simulink model "core_attitude"  (R2022b)
settings: Solver=ode4  StartTime=0.0  StopTime=100  FixedStep=0.1  RelTol=1e-3
values from neighbouring files (symbols this model uses):
  A0 = diag([1 1 1])    [LAB_04_17_OCT_MAT_KIN.m]    (also in LAB_05_24_OCT_MAT_KIN_COSDIR.m; LAB_06.m = A_target_fun(0); core_attitude_test.m = eye(3,3); lab_07_MAT.m)
  I = [Ix 0 0 ... (first row only)    [LAB_03_3_OCT_MAT_EUL_2_VERIFICATION.m]    (also in LAB_03_3_OCT_MAT_EUL_DOUBLESPIN.m = diag([Ix, Iy, Iz]); LAB_03_3_OCT_MAT_EUL_SPINAXIS.m = diag([Ix, Iy, Iz]); LAB_03_3_OCT_MAT_EUL_VECT.m; LAB_04_17_OCT_MAT_KIN.m)
  om_0 = [om_x0, om_y0, om_z0]    [LAB_03_3_OCT_MAT_EUL.m]    (also in LAB_03_3_OCT_MAT_EUL_2_VERIFICATION.m = [om_x0; om_y0; om_z0]; LAB_03_3_OCT_MAT_EUL_DOUBLESPIN.m = [om_x0; om_y0; om_z0]; LAB_03_3_OCT_MAT_EUL_SPINAXIS.m = [om_x0; om_y0; om_z0]; LAB_03_3_OCT_MAT_EUL_VECT.m = [om_x0; om_y0; om_z0])
  q0 = [0, 0, 0, 1]'    [LAB_04_17_OCT_MAT_KIN.m]    (also in core_attitude_test.m = [0;0;0;1])
libraries: sharedutil x2, matrix_library x1
settings Model: Creator=maria  LastModifiedBy=maria

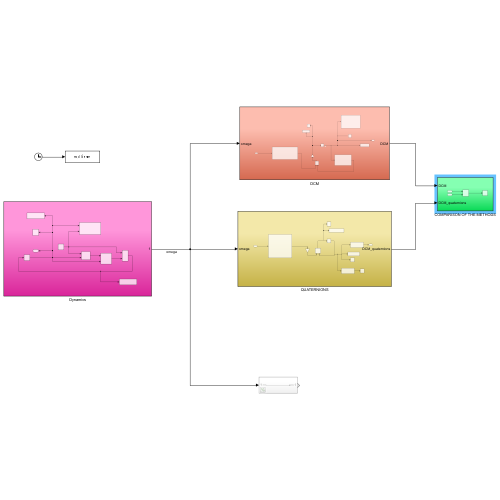
[thumbnail: Simulink's stored preview of the top-level diagram]
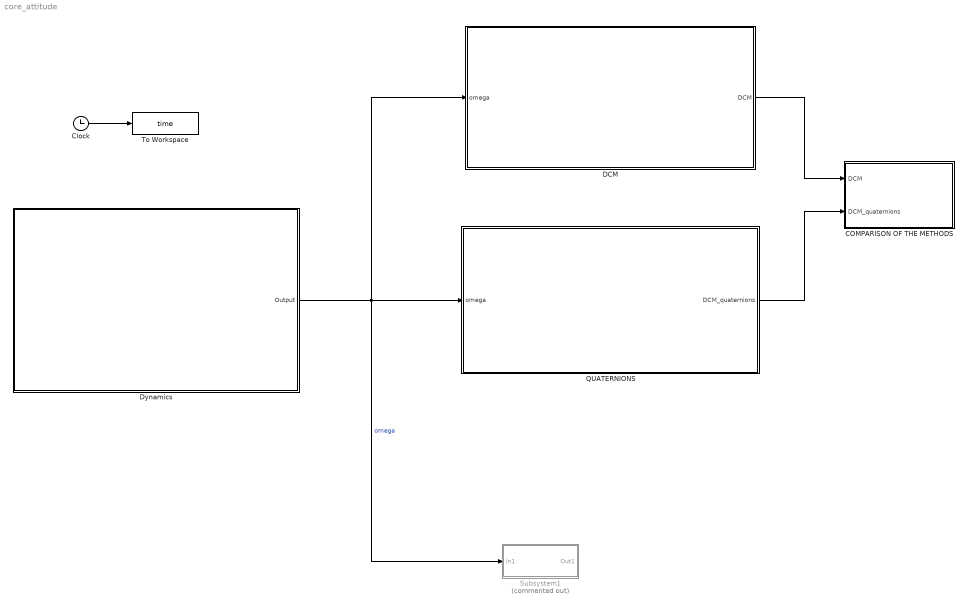
== system core_attitude ==
  COMPARISON OF THE METHODS : Subsystem
  Clock : Clock
  DCM : Subsystem
  Dynamics : Subsystem
  QUATERNIONS : Subsystem
  Subsystem1 : Subsystem  Commented=on
  To Workspace : ToWorkspace  VariableName=time  SaveFormat=Timeseries  SampleTime=-1
  wires:
  Clock/1 -> To Workspace/1
  Dynamics/1(Output) -> DCM/1(omega), QUATERNIONS/1(omega), Subsystem1/1(In1)  "omega"
  DCM/1(DCM) -> COMPARISON OF THE METHODS/1(DCM)
  QUATERNIONS/1(DCM_quaternions) -> COMPARISON OF THE METHODS/2(DCM_quaternions)

== system core_attitude/COMPARISON OF THE METHODS ==
  DCM : Inport
  DCM_quaternions : Inport  Port=2
  Scope : Scope
  Sum : Sum  Inputs=+-
  wires:
  DCM/1 -> Sum/1
  DCM_quaternions/1 -> Sum/2
  Sum/1 -> Scope/1

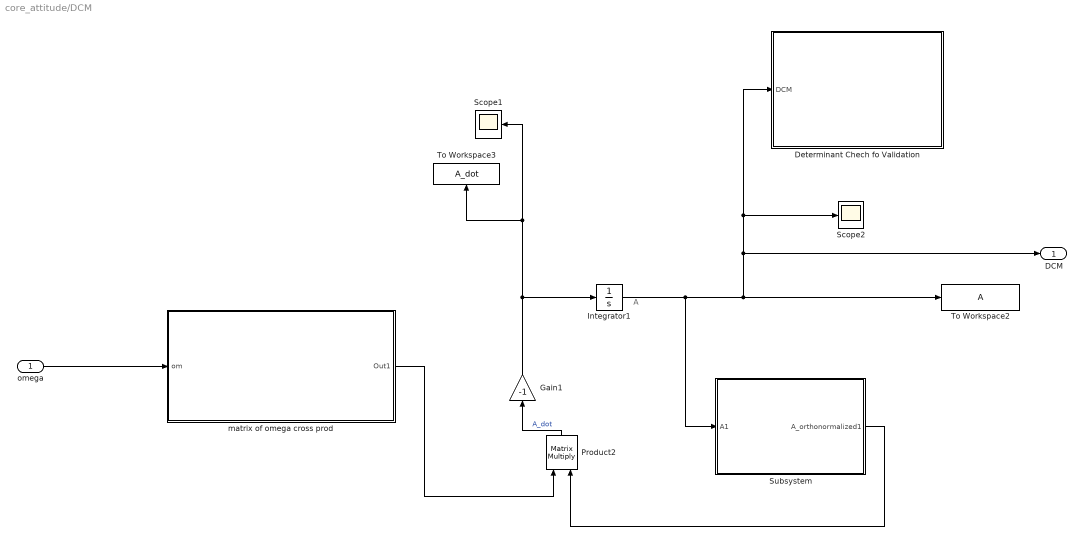
== system core_attitude/DCM ==
  note: A
  omega : Inport
  Determinant Chech fo Validation : Subsystem
  Gain1 : Gain  Gain=-1
  Integrator1 : Integrator  InitialCondition=A0
  Product2 : Product  Multiplication=Matrix(*)
  Scope1 : Scope
  Scope2 : Scope
  Subsystem : Subsystem
  To Workspace2 : ToWorkspace  VariableName=A  SampleTime=-1
  To Workspace3 : ToWorkspace  VariableName=A_dot  SampleTime=-1
  matrix of omega cross prod : Subsystem
  DCM : Outport
  wires:
  Integrator1/1 -> Subsystem/1(A1), Scope2/1, Determinant Chech fo Validation/1(DCM), DCM/1, To Workspace2/1
  matrix of omega cross prod/1(Out1) -> Product2/1
  Product2/1 -> Gain1/1  "A_dot"
  omega/1 -> matrix of omega cross prod/1(om)
  Gain1/1 -> Integrator1/1, To Workspace3/1, Scope1/1
  Subsystem/1(A_orthonormalized1) -> Product2/2

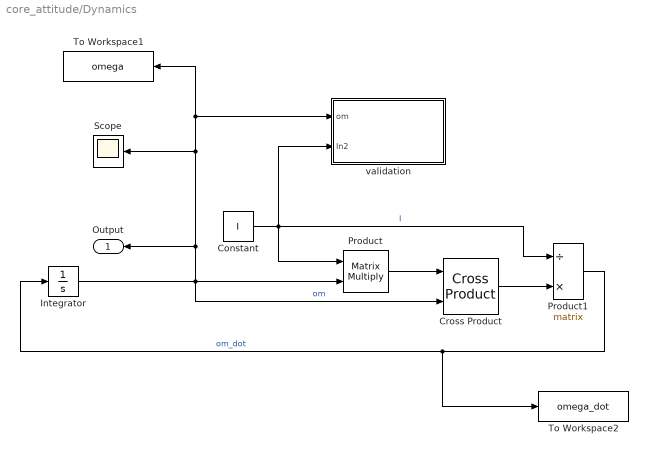
== system core_attitude/Dynamics ==
  Constant : Constant  Value=I
  Cross Product : matrix_library/Cross Product
  Integrator : Integrator  InitialCondition=om_0
  Product : Product  Multiplication=Matrix(*)
  Product1 : Product  Inputs=/*  Multiplication=Matrix(*)
  Scope : Scope
  To Workspace1 : ToWorkspace  VariableName=omega  SampleTime=-1
  To Workspace2 : ToWorkspace  VariableName=omega_dot  SampleTime=-1
  validation : Subsystem
  Output : Outport
  wires:
  Product1/1 -> To Workspace2/1, Integrator/1  "om_dot"
  Integrator/1 -> Product/2, Cross Product/2, validation/1(om), To Workspace1/1, Scope/1, Output/1  "om"
  Cross Product/1 -> Product1/2
  Constant/1 -> Product1/1, Product/1, validation/2(In2)  "I"
  Product/1 -> Cross Product/1

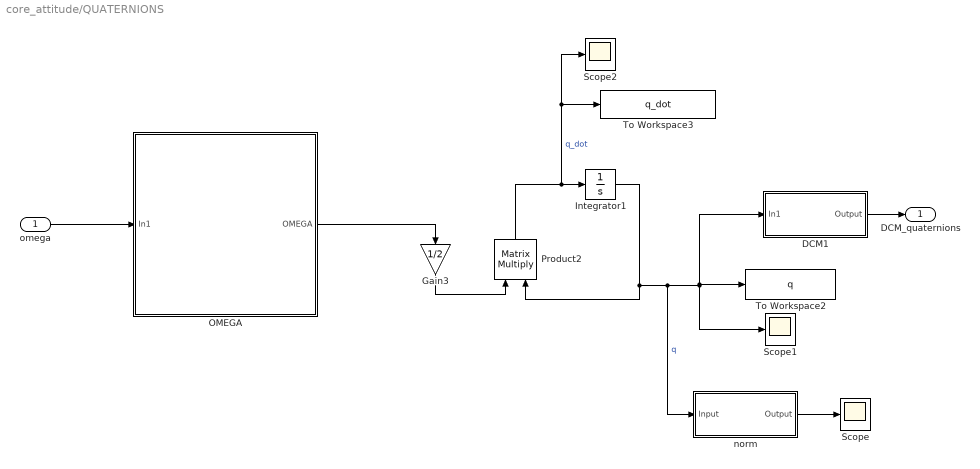
== system core_attitude/QUATERNIONS ==
  omega : Inport
  DCM1 : Subsystem
  Gain3 : Gain  Gain=1/2
  Integrator1 : Integrator  InitialCondition=q0
  OMEGA : Subsystem
  Product2 : Product  Multiplication=Matrix(*)
  Scope : Scope
  Scope1 : Scope
  Scope2 : Scope
  To Workspace2 : ToWorkspace  VariableName=q  SaveFormat=Timeseries  SampleTime=-1
  To Workspace3 : ToWorkspace  VariableName=q_dot  SaveFormat=Timeseries  SampleTime=-1
  norm : Subsystem
  DCM_quaternions : Outport
  wires:
  Gain3/1 -> Product2/1
  OMEGA/1(OMEGA) -> Gain3/1
  Product2/1 -> Scope2/1, To Workspace3/1, Integrator1/1  "q_dot"
  Integrator1/1 -> Product2/2, norm/1(Input), DCM1/1(In1), To Workspace2/1, Scope1/1  "q"
  omega/1 -> OMEGA/1(In1)
  DCM1/1(Output) -> DCM_quaternions/1
  norm/1(Output) -> Scope/1

== system core_attitude/Subsystem1 ==
  In1 : Inport
  Out1 : Outport
  wires:
  In1/1 -> Out1/1

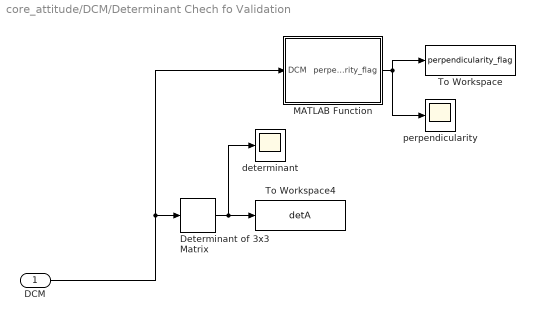
== system core_attitude/DCM/Determinant Chech fo Validation ==
  DCM : Inport
  Determinant of 3x3 Matrix : sharedutil/Determinant of 3x3 Matrix  aMode=aMode
      settings: LibrarySourceBlock=|
      | aerolibutil/Determinant of
      | 3x3 Matrix
  MATLAB Function : MATLAB Function  TreatAsAtomicUnit=on
  To Workspace : ToWorkspace  VariableName=perpendicularity_flag  SampleTime=-1
  To Workspace4 : ToWorkspace  VariableName=detA  SampleTime=-1
  determinant : Scope
  perpendicularity : Scope
  wires:
  Determinant of 3x3 Matrix/1 -> determinant/1, To Workspace4/1
  DCM/1 -> MATLAB Function/1(DCM), Determinant of 3x3 Matrix/1
  MATLAB Function/1(perpendicularity_flag) -> To Workspace/1, perpendicularity/1

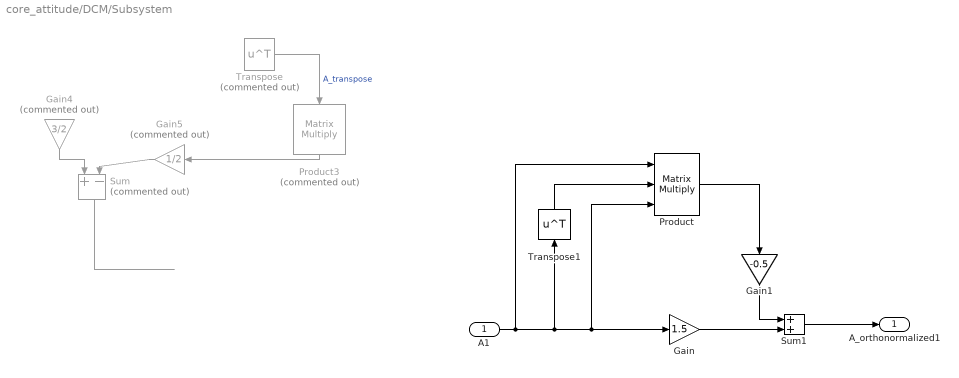
== system core_attitude/DCM/Subsystem ==
  A1 : Inport
  Gain : Gain  Gain=1.5
  Gain1 : Gain  Gain=-0.5
  Gain4 : Gain  Commented=on  Gain=3/2
  Gain5 : Gain  Commented=on  Gain=1/2
  Product : Product  Inputs=3  Multiplication=Matrix(*)
  Product3 : Product  Commented=on  Inputs=3  Multiplication=Matrix(*)
  Sum : Sum  Commented=on  Inputs=+-
  Sum1 : Sum
  Transpose : Math  Commented=on  Operator=transpose
  Transpose1 : Math  Operator=transpose
  A_orthonormalized1 : Outport
  wires:
  Sum/1 -> ?
  Gain5/1 -> Sum/2
  Product3/1 -> Gain5/1
  Transpose/1 -> Product3/2  "A_transpose"
  Gain4/1 -> Sum/1
  A1/1 -> Product/1, Transpose1/1, Product/3, Gain/1
  Gain/1 -> Sum1/2
  Sum1/1 -> A_orthonormalized1/1
  Gain1/1 -> Sum1/1
  Product/1 -> Gain1/1
  Transpose1/1 -> Product/2

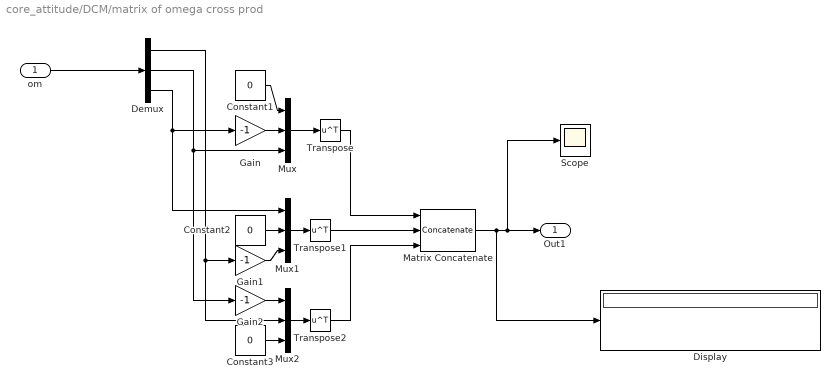
== system core_attitude/DCM/matrix of omega cross prod ==
  om : Inport
  Constant1 : Constant  Value=0
  Constant2 : Constant  Value=0
  Constant3 : Constant  Value=0
  Demux : Demux  Outputs=3
  Display : Display
  Gain : Gain  Gain=-1
  Gain1 : Gain  Gain=-1
  Gain2 : Gain  Gain=-1
  Matrix Concatenate : Concatenate  NumInputs=3  Mode=Multidimensional array
  Mux : Mux  Inputs=3
  Mux1 : Mux  Inputs=3
  Mux2 : Mux  Inputs=3
  Scope : Scope
  Transpose : Math  Operator=transpose
  Transpose1 : Math  Operator=transpose
  Transpose2 : Math  Operator=transpose
  Out1 : Outport
  wires:
  Matrix Concatenate/1 -> Display/1, Scope/1, Out1/1
  Demux/1 -> Gain1/1, Mux2/2
  Mux1/1 -> Transpose1/1
  Constant3/1 -> Mux2/3
  Gain/1 -> Mux/2
  Gain2/1 -> Mux2/1
  Constant1/1 -> Mux/1
  Demux/3 -> Gain/1, Mux1/1
  Demux/2 -> Mux/3, Gain2/1
  Mux/1 -> Transpose/1
  Gain1/1 -> Mux1/3
  Mux2/1 -> Transpose2/1
  Constant2/1 -> Mux1/2
  om/1 -> Demux/1
  Transpose/1 -> Matrix Concatenate/1
  Transpose1/1 -> Matrix Concatenate/2
  Transpose2/1 -> Matrix Concatenate/3

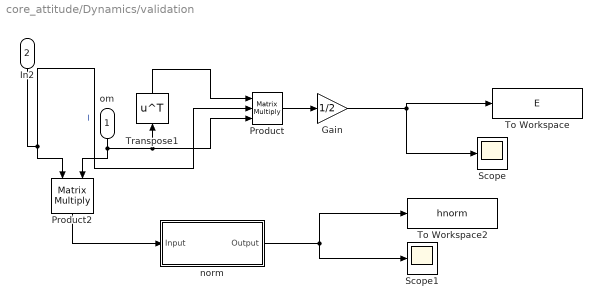
== system core_attitude/Dynamics/validation ==
  om : Inport
  In2 : Inport  Port=2
  Gain : Gain  Gain=1/2
  Product : Product  Inputs=3  Multiplication=Matrix(*)
  Product2 : Product  Multiplication=Matrix(*)
  Scope : Scope
  Scope1 : Scope
  To Workspace : ToWorkspace  VariableName=E  SampleTime=-1
  To Workspace2 : ToWorkspace  VariableName=hnorm  SampleTime=-1
  Transpose1 : Math  Operator=transpose
  norm : Subsystem
  wires:
  Product2/1 -> norm/1(Input)
  norm/1(Output) -> To Workspace2/1, Scope1/1
  om/1 -> Transpose1/1, Product/3, Product2/2
  In2/1 -> Product/2, Product2/1  "I"
  Transpose1/1 -> Product/1
  Product/1 -> Gain/1
  Gain/1 -> Scope/1, To Workspace/1

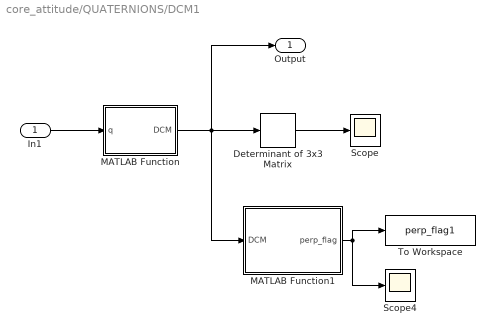
== system core_attitude/QUATERNIONS/DCM1 ==
  In1 : Inport
  Determinant of 3x3 Matrix : sharedutil/Determinant of 3x3 Matrix  aMode=aMode
      settings: LibrarySourceBlock=|
      | aerolibutil/Determinant of
      | 3x3 Matrix
  MATLAB Function : MATLAB Function  TreatAsAtomicUnit=on
  MATLAB Function1 : MATLAB Function  TreatAsAtomicUnit=on
  Scope : Scope
  Scope4 : Scope
  To Workspace : ToWorkspace  VariableName=perp_flag1  SampleTime=-1
  Output : Outport
  wires:
  In1/1 -> MATLAB Function/1(q)
  MATLAB Function/1(DCM) -> Output/1, Determinant of 3x3 Matrix/1, MATLAB Function1/1(DCM)
  Determinant of 3x3 Matrix/1 -> Scope/1
  MATLAB Function1/1(perp_flag) -> To Workspace/1, Scope4/1

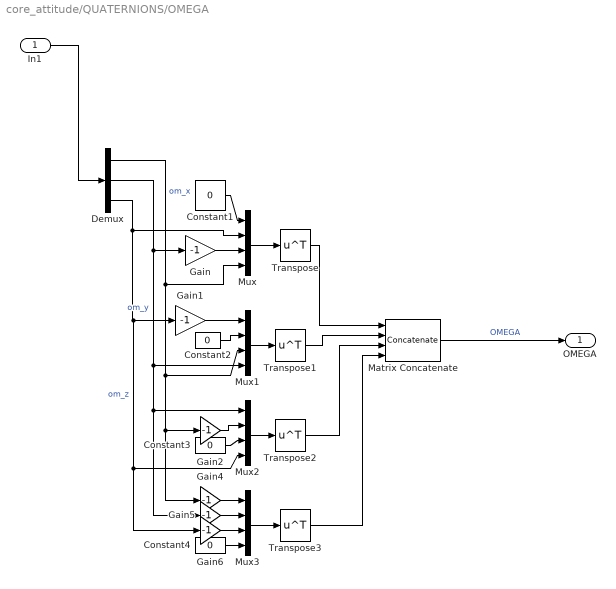
== system core_attitude/QUATERNIONS/OMEGA ==
  In1 : Inport
  Constant{1..4} (4 alike) : Constant  Value=0
  Demux : Demux  Outputs=3
  Gain{,1..2,4..6} (6 alike) : Gain  Gain=-1
  Matrix Concatenate : Concatenate  NumInputs=4  Mode=Multidimensional array
  Mux{,1..3} (4 alike) : Mux
  Transpose{,1..3} (4 alike) : Math  Operator=transpose
  OMEGA : Outport
  wires:
  Mux/1 -> Transpose/1
  Constant2/1 -> Mux1/2
  Matrix Concatenate/1 -> OMEGA/1  "OMEGA"
  Constant4/1 -> Mux3/4
  Mux2/1 -> Transpose2/1
  Constant1/1 -> Mux/1
  Constant3/1 -> Mux2/3
  Demux/3 -> Mux/2, Gain6/1, Mux2/4, Gain1/1  "om_z"
  Gain2/1 -> Mux2/2
  Demux/2 -> Gain5/1, Mux2/1, Mux1/4, Gain/1  "om_y"
  Gain6/1 -> Mux3/3
  Mux3/1 -> Transpose3/1
  Demux/1 -> Mux/4, Mux1/3, Gain4/1, Gain2/1  "om_x"
  Gain4/1 -> Mux3/1
  Gain/1 -> Mux/3
  Gain1/1 -> Mux1/1
  Gain5/1 -> Mux3/2
  In1/1 -> Demux/1
  Transpose/1 -> Matrix Concatenate/1
  Mux1/1 -> Transpose1/1
  Transpose1/1 -> Matrix Concatenate/2
  Transpose2/1 -> Matrix Concatenate/3
  Transpose3/1 -> Matrix Concatenate/4

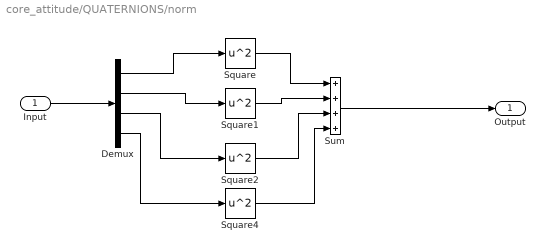
== system core_attitude/QUATERNIONS/norm ==
  Input : Inport
  Demux : Demux
  Square{,1..2,4} (4 alike) : Math  Operator=square
  Sum : Sum  Inputs=++++
  Output : Outport
  wires:
  Square/1 -> Sum/1
  Square1/1 -> Sum/2
  Square2/1 -> Sum/3
  Input/1 -> Demux/1
  Sum/1 -> Output/1
  Demux/1 -> Square/1
  Demux/2 -> Square1/1
  Demux/3 -> Square2/1
  Demux/4 -> Square4/1
  Square4/1 -> Sum/4

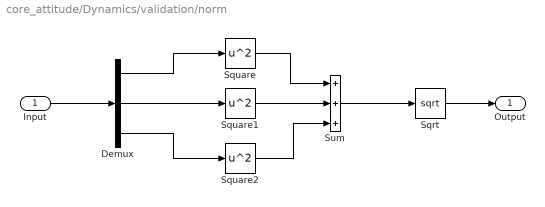
== system core_attitude/Dynamics/validation/norm ==
  Input : Inport
  Demux : Demux  Outputs=3
  Sqrt : Sqrt
  Square : Math  Operator=square
  Square1 : Math  Operator=square
  Square2 : Math  Operator=square
  Sum : Sum  Inputs=+++
  Output : Outport
  wires:
  Square/1 -> Sum/1
  Square1/1 -> Sum/2
  Square2/1 -> Sum/3
  Sum/1 -> Sqrt/1
  Input/1 -> Demux/1
  Sqrt/1 -> Output/1
  Demux/1 -> Square/1
  Demux/2 -> Square1/1
  Demux/3 -> Square2/1

== matlab function core_attitude/DCM/Determinant Chech fo Validation/MATLAB Function ==
  data: DCM input; perpendicularity_flag output
function perpendicularity_flag = fcn(DCM)


perpendicularity_flag =zeros(3,1);

    x   = DCM(1,:);
    y   = DCM(2,:);
    z   = DCM(3,:);

    perpendicularity_flag(1)=dot(x,y);
    perpendicularity_flag(2)=dot(x,z);
    perpendicularity_flag(3)=dot(z,y);

end

== matlab function core_attitude/QUATERNIONS/DCM1/MATLAB Function1 ==
  data: DCM input; perp_flag output
function perp_flag = fcn(DCM)


perp_flag =zeros(3,1);

    x   = DCM(1,:);
    y   = DCM(2,:);
    z   = DCM(3,:);

    perp_flag(1)=dot(x,y);
    perp_flag(2)=dot(x,z);
    perp_flag(3)=dot(z,y);

end

== matlab function core_attitude/QUATERNIONS/DCM1/MATLAB Function ==
  data: q input; DCM output
function DCM = fcn(q)

q1 = q(1);
q2 = q(2);
q3 = q(3);
q4 = q(4);

DCM = [q1^2-q2^2-q3^2+q4^2, 2*(q1*q2+q3*q4), 2*(q1*q3-q2*q4);
        2*(q1*q2-q3*q4), -q1^2+q2^2-q3^2+q4^2, 2*(q2*q3+q1*q4);
        2*(q1*q3+q2*q4), 2*(q2*q3-q1*q4), -q1^2-q2^2+q3^2+q4^2];

end
